simulink model "simulinkObservador2017"  (R2017a)
settings: Solver=VariableStepAuto  StartTime=0.0  StopTime=5  FixedStep=0.000001  RelTol=1e-3
values from neighbouring files (symbols this model uses):
  Ad = [1 0 0 0 0.02 0.9238096 0 0 0 0.1756458 1 -3.08956 ... (16 elements, 4x4)]    [medicion_obs.mat]    (also in observador_completo.m = eye(4) + Ts*A; realimentacion_feed.m = eye(4) + Ts*A; realimentacion_integral.m = eye(4) + Ts*A; realimentacion_sin_feed.m = eye(4) + Ts*A)
  Bd = [0 0 0 1.2978]    [medicion_obs.mat]    (also in observador_completo.m = B*Ts; realimentacion_feed.m = B*Ts; realimentacion_integral.m = B*Ts; realimentacion_sin_feed.m = B*Ts)
  Ld = [1.13488978473  3.3327939085e-15; 13.9805864099  0.1756458; 1.20460366503e-16  0.79628018473; 9.02712676923e-16  -1.30043928872]    [medicion_obs.mat]    (also in observador_completo.m = place(Ad',Cd',polos_discretos)')
libraries: simulink x1
settings Model: Creator=PC  LastModifiedBy=q
settings DataIOCC: ReturnWorkspaceOutputs=on
settings SFSimCC: SimUseLocalCustomCode=on
settings RTWCC: RTWUseLocalCustomCode=on

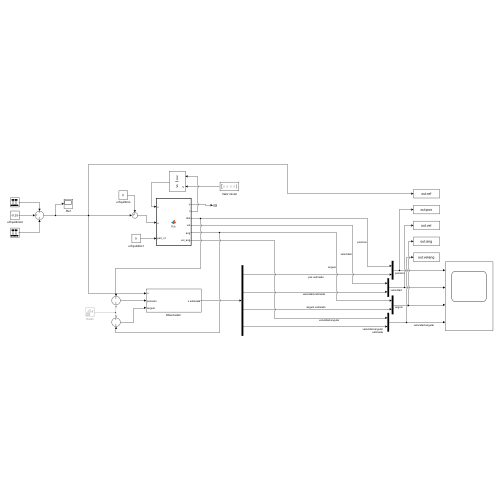
[thumbnail: Simulink's stored preview of the top-level diagram]
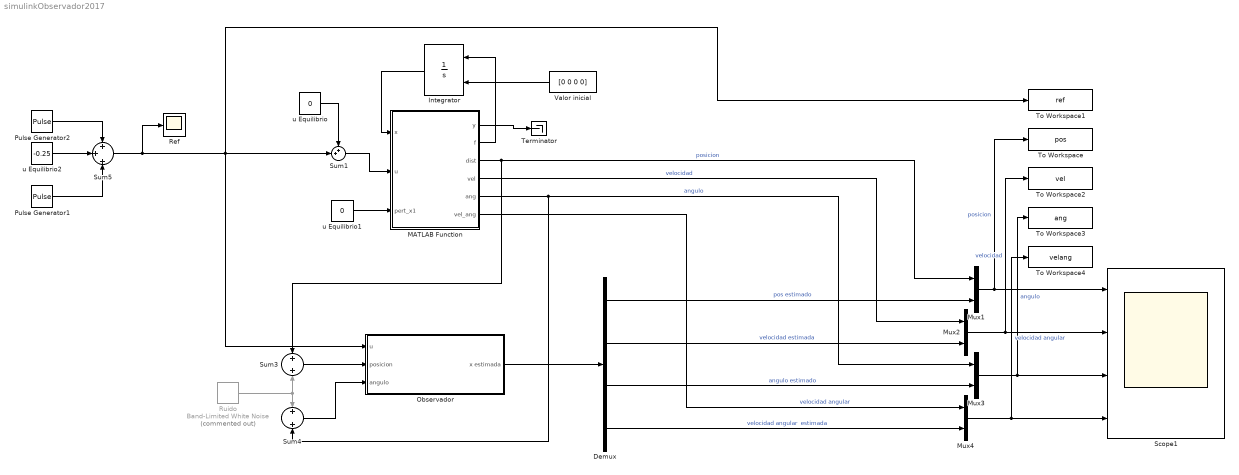
== system simulinkObservador2017 ==
  Demux : Demux
  Integrator : Integrator  InitialConditionSource=external
  MATLAB Function : MATLAB Function  TreatAsAtomicUnit=on
  Mux{1..4} (4 alike) : Mux  Inputs=2
  "Observador " : Subsystem
  Pulse Generator1 : DiscretePulseGenerator  Amplitude=0.25  Period=100  PulseWidth=60  PhaseDelay=40  SampleTime=0.02
  Pulse Generator2 : DiscretePulseGenerator  Amplitude=0.5  Period=100  PulseWidth=20  SampleTime=0.02
  Ref : Scope
  Ruido : simulink/Sources/Band-Limited White Noise  Commented=on  Cov=0.000005  Ts=0.02  seed=[23341]
  Scope1 : Scope  NumInputPorts=4
  Sum1 : Sum  Inputs=++|
  Sum3 : Sum  Inputs=+|+
  Sum4 : Sum  Inputs=+|+
  Sum5 : Sum  Inputs=+|+|+
  Terminator : Terminator
  To Workspace : ToWorkspace  VariableName=pos  SampleTime=0.02
      settings: Save2DSignal=2-D array (concatenate along first dimension)
  To Workspace1 : ToWorkspace  VariableName=ref  SampleTime=0.02
      settings: Save2DSignal=2-D array (concatenate along first dimension)
  To Workspace2 : ToWorkspace  VariableName=vel  SampleTime=0.02
      settings: Save2DSignal=2-D array (concatenate along first dimension)
  To Workspace3 : ToWorkspace  VariableName=ang  SampleTime=0.02
      settings: Save2DSignal=2-D array (concatenate along first dimension)
  To Workspace4 : ToWorkspace  VariableName=velang  SampleTime=0.02
      settings: Save2DSignal=2-D array (concatenate along first dimension)
  Valor inicial : Constant  Value=[0 0 0 0]
  u Equilibrio : Constant  Value=0
  u Equilibrio1 : Constant  Value=0
  u Equilibrio2 : Constant  Value=-0.25  SampleTime=0.02
  wires:
  Valor inicial/1 -> Integrator/2
  MATLAB Function/2(f) -> Integrator/1
  u Equilibrio/1 -> Sum1/1
  Sum1/1 -> MATLAB Function/2(u)
  Integrator/1 -> MATLAB Function/1(x)
  MATLAB Function/6(vel_ang) -> Mux4/1  "velocidad angular"
  Demux/4 -> Mux4/2  "velocidad angular  estimada"
  Mux1/1 -> To Workspace/1, Scope1/1  "posicion"
  Demux/1 -> Mux1/2  "pos estimado"
  Mux2/1 -> To Workspace2/1, Scope1/2  "velocidad"
  Mux4/1 -> Scope1/4, To Workspace4/1  "velocidad angular"
  Demux/2 -> Mux2/2  "velocidad estimada"
  Demux/3 -> Mux3/2  "angulo estimado"
  MATLAB Function/5(ang) -> Mux3/1, Sum4/2  "angulo"
  Mux3/1 -> To Workspace3/1, Scope1/3  "angulo"
  MATLAB Function/4(vel) -> Mux2/1  "velocidad"
  MATLAB Function/3(dist) -> Sum3/1, Mux1/1  "posicion"
  MATLAB Function/1(y) -> Terminator/1
  u Equilibrio1/1 -> MATLAB Function/3(pert_x1)
  "Observador "/1(x estimada) -> Demux/1
  Ruido/1 -> Sum3/2, Sum4/1
  Sum4/1 -> "Observador "/3(angulo)
  Sum3/1 -> "Observador "/2(posicion)
  Pulse Generator2/1 -> Sum5/1
  u Equilibrio2/1 -> Sum5/2
  Pulse Generator1/1 -> Sum5/3
  Sum5/1 -> Ref/1, To Workspace1/1, Sum1/2, "Observador "/1(u)

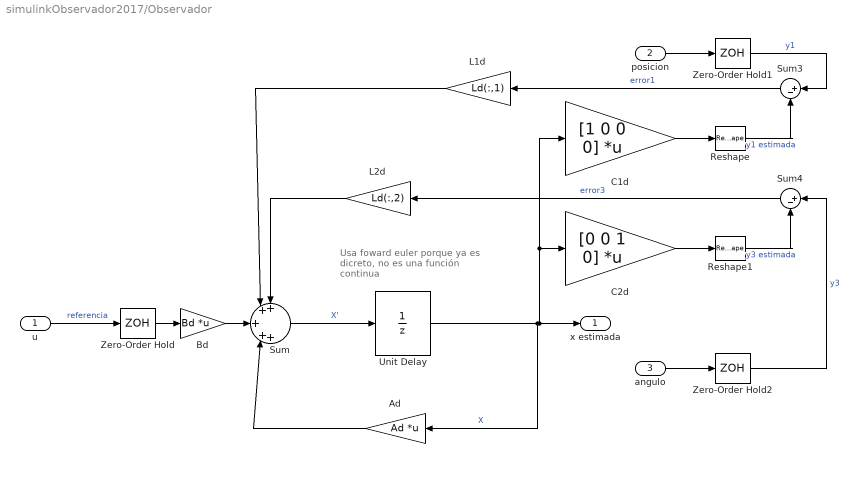
== system simulinkObservador2017/Observador  ==
  note: Usa foward euler porque ya es dicreto, no es una función continua
  u : Inport
  posicion : Inport  Port=2
  angulo : Inport  Port=3
  Ad : Gain  Gain=Ad  Multiplication=Matrix(K*u)
  Bd : Gain  Gain=Bd  Multiplication=Matrix(K*u)
  C1d : Gain  Gain=[1 0 0 0]  Multiplication=Matrix(K*u)
  C2d : Gain  Gain=[0 0 1 0]  Multiplication=Matrix(K*u)
  L1d : Gain  Gain=Ld(:,1)
  L2d : Gain  Gain=Ld(:,2)
  Reshape : Reshape
  Reshape1 : Reshape  OutputDimensions=[1]
  Sum : Sum  Inputs=++|+|++
  Sum3 : Sum  Inputs=|+-
  Sum4 : Sum  Inputs=|+-
  Unit Delay : UnitDelay  SampleTime=0.02  HasFrameUpgradeWarning=on
  Zero-Order Hold : ZeroOrderHold  SampleTime=0.02
  Zero-Order Hold1 : ZeroOrderHold  SampleTime=0.02
  Zero-Order Hold2 : ZeroOrderHold  SampleTime=0.02
  x estimada : Outport
  wires:
  u/1 -> Zero-Order Hold/1  "referencia"
  Ad/1 -> Sum/4
  Zero-Order Hold/1 -> Bd/1
  Bd/1 -> Sum/3
  Sum/1 -> Unit Delay/1  "X'"
  Unit Delay/1 -> C2d/1, C1d/1, x estimada/1, Ad/1  "X"
  C1d/1 -> Reshape/1
  posicion/1 -> Zero-Order Hold1/1
  angulo/1 -> Zero-Order Hold2/1
  C2d/1 -> Reshape1/1
  Zero-Order Hold1/1 -> Sum3/1  "y1"
  Reshape1/1 -> Sum4/2  "y3 estimada"
  Reshape/1 -> Sum3/2  "y1 estimada"
  Zero-Order Hold2/1 -> Sum4/1  "y3"
  Sum3/1 -> L1d/1  "error1"
  Sum4/1 -> L2d/1  "error3"
  L2d/1 -> Sum/1
  L1d/1 -> Sum/2

== matlab function simulinkObservador2017/MATLAB Function ==
  data: x input; u input; y output; f output; pert_x1 input; dist output; vel output; ang output; vel_ang output
function [y, f,dist,vel,ang,vel_ang] = fcn(x, u, pert_x1)
    
    g = 9.81; %kg m/s2
    m = 0.047; %kg
    kv = 0.2;
    R = 0.02;
    mr = 0.00275;
    J = 0.5*4*mr*power(R,2);
    
    x(1) = x(1) + pert_x1;

    %Dinamica
    f1 = x(2);
    f2 = (m*g*sin(x(3)) - kv * x(2)) * 1/(m + (J/power(R,2)));
    f3 = x(4);
    f4 = -20.73 * x(4) - 154.47*x(3) + u * 64.89;

    y = x(1);
    f = [f1 f2 f3 f4];
    dist=x(1);
    vel=x(2);
    ang=x(3);
    vel_ang=x(4);
end
